simulink model "emulation_method"  (R2020b)
settings: Solver=ode45  StartTime=0.0  StopTime=5  FixedStep=0.0001  RelTol=1e-3
undefined symbols (not defined in the file): ctrl, daq, degs2rpm, denHwa, denHws, DiscIntNeverNeededParam, drv, gbox, K_w, mld, mot, numHwa, numHws, rads2rpm, sens, step_size, T, tau_hat, Tl
settings Model: Creator=gioel  LastModifiedBy=gioel
settings DataIOCC: ReturnWorkspaceOutputs=off

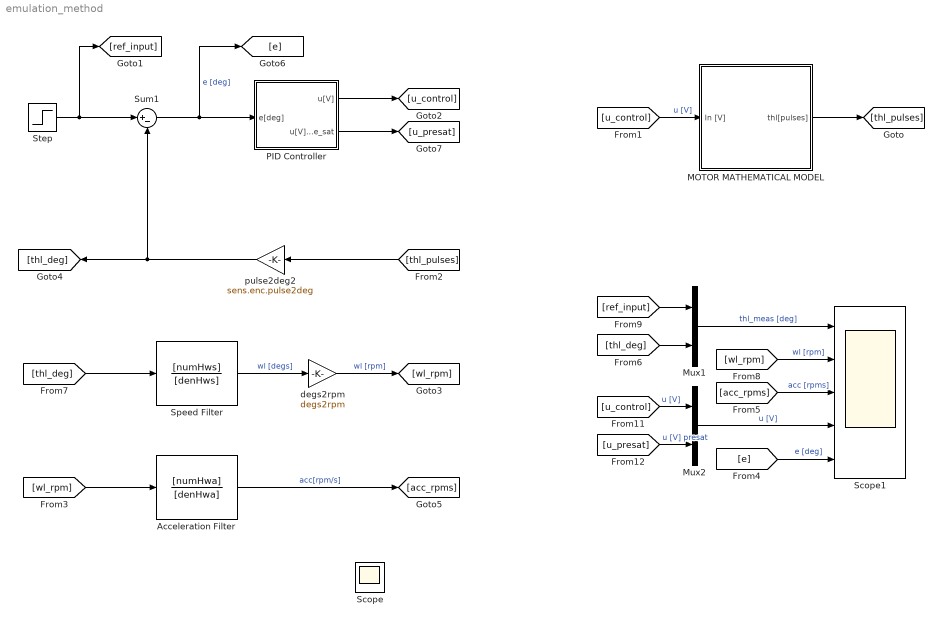
== system emulation_method ==
  Acceleration Filter : TransferFcn  Numerator=[numHwa]  Denominator=[denHwa]
  MOTOR MATHEMATICAL MODEL : Subsystem
  Mux1 : Mux  Inputs=2
  Mux2 : Mux  Inputs=2
  PID Controller : Subsystem
  Scope1 : Scope  NumInputPorts=5
  Speed Filter : TransferFcn  Numerator=[numHws]  Denominator=[denHws]
  Step : Step  After=step_size  SampleTime=0
  Sum1 : Sum  Inputs=|+-
  degs2rpm : Gain  Gain=degs2rpm
  pulse2deg2 : Gain  Gain=sens.enc.pulse2deg
  Scope : Scope
  wires:
  Sum1/1 -> [e], PID Controller/1(e[deg])  "e [deg]"
  Step/1 -> Sum1/1, [ref_input]
  PID Controller/1(u[V]) -> [u_control]
  Mux1/1 -> Scope1/1  "thl_meas [deg]"
  MOTOR MATHEMATICAL MODEL/1(thl[pulses]) -> [thl_pulses]
  degs2rpm/1 -> [wl_rpm]  "wl [rpm]"
  [thl_deg] -> Mux1/2
  [acc_rpms] -> Scope1/3  "acc [rpms]"
  [u_control] -> MOTOR MATHEMATICAL MODEL/1(In [V])  "u [V]"
  Mux2/1 -> Scope1/4  "u [V]"
  Speed Filter/1 -> degs2rpm/1  "wl [degs]"
  [wl_rpm] -> Scope1/2  "wl [rpm]"
  [wl_rpm] -> Acceleration Filter/1
  [thl_deg] -> Speed Filter/1
  [ref_input] -> Mux1/1
  Acceleration Filter/1 -> [acc_rpms]  "acc[rpm/s]"
  pulse2deg2/1 -> Sum1/2, [thl_deg]
  [thl_pulses] -> pulse2deg2/1
  [e] -> Scope1/5  "e [deg]"
  PID Controller/2(u[V] pre_sat) -> [u_presat]
  [u_control] -> Mux2/1  "u [V]"
  [u_presat] -> Mux2/2  "u [V] presat"

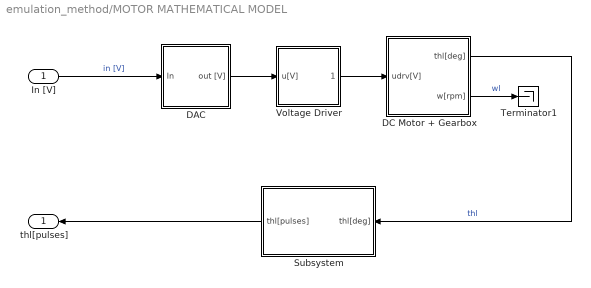
== system emulation_method/MOTOR MATHEMATICAL MODEL ==
  In [V] : Inport
  DAC : Subsystem
  DC Motor + Gearbox : Subsystem
  Subsystem : Subsystem
  Terminator1 : Terminator
  Voltage Driver : Subsystem
  thl[pulses] : Outport
  wires:
  In [V]/1 -> DAC/1(In)  "in [V]"
  DC Motor + Gearbox/1(thl[deg]) -> Subsystem/1(thl[deg])  "thl"
  DAC/1(out [V]) -> Voltage Driver/1(u[V])
  DC Motor + Gearbox/2(w[rpm]) -> Terminator1/1  "wl"
  Subsystem/1(thl[pulses]) -> thl[pulses]/1
  Voltage Driver/1(udrv[V]) -> DC Motor + Gearbox/1(udrv[V])

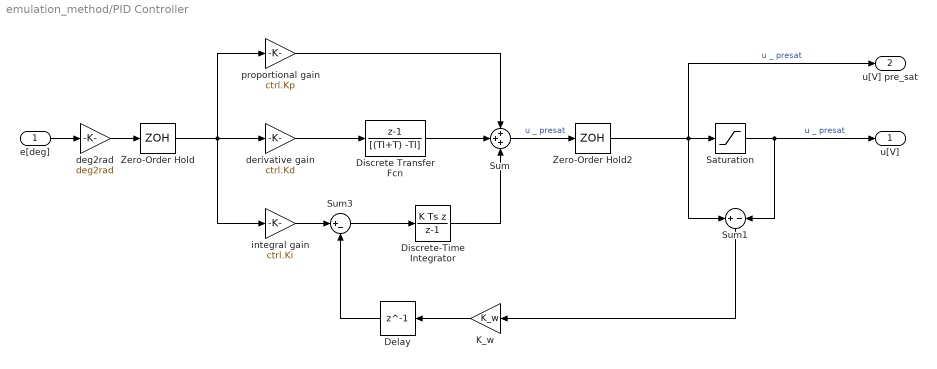
== system emulation_method/PID Controller ==
  e[deg] : Inport
  Delay : Delay  DelayLength=1  InitialCondition=0  SampleTime=T
  Discrete Transfer Fcn : DiscreteTransferFcn  Numerator=[1 -1]  Denominator=[(Tl+T) -Tl]  SampleTime=T
  Discrete-Time Integrator : DiscreteIntegrator  IntegratorMethod=Integration: Backward Euler  SampleTime=T  ICPrevOutput=DiscIntNeverNeededParam  ICPrevScaledInput=DiscIntNeverNeededParam
  "K_w " : Gain  Gain=K_w
  Saturation : Saturate  UpperLimit=10  LowerLimit=-10
  Sum : Sum  Inputs=+++
  Sum1 : Sum  Inputs=+|-
  Sum3 : Sum  Inputs=|+-
  Zero-Order Hold : ZeroOrderHold  SampleTime=T
  Zero-Order Hold2 : ZeroOrderHold  SampleTime=T
  deg2rad : Gain  Gain=deg2rad
  derivative gain : Gain  Gain=ctrl.Kd
  integral gain : Gain  Gain=ctrl.Ki
  proportional gain : Gain  Gain=ctrl.Kp
  u[V] : Outport
  u[V] pre_sat : Outport  Port=2
  wires:
  proportional gain/1 -> Sum/1
  e[deg]/1 -> deg2rad/1
  deg2rad/1 -> Zero-Order Hold/1
  Zero-Order Hold/1 -> integral gain/1, derivative gain/1, proportional gain/1
  derivative gain/1 -> Discrete Transfer Fcn/1
  Discrete Transfer Fcn/1 -> Sum/2
  Discrete-Time Integrator/1 -> Sum/3
  Sum1/1 -> "K_w "/1
  integral gain/1 -> Sum3/1
  Sum3/1 -> Discrete-Time Integrator/1
  "K_w "/1 -> Delay/1
  Delay/1 -> Sum3/2
  Sum/1 -> Zero-Order Hold2/1  "u _ presat"
  Saturation/1 -> u[V]/1, Sum1/2  "u _ presat"
  Zero-Order Hold2/1 -> u[V] pre_sat/1, Sum1/1, Saturation/1  "u _ presat"

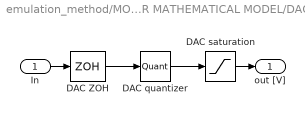
== system emulation_method/MOTOR MATHEMATICAL MODEL/DAC ==
  In : Inport
  DAC quantizer : Quantizer  QuantizationInterval=daq.dac.q
  DAC saturation : Saturate  UpperLimit=daq.dac.fs  LowerLimit=-daq.dac.fs
  DAC ZOH : ZeroOrderHold  SampleTime=0.001
  out [V] : Outport
  wires:
  DAC saturation/1 -> out [V]/1
  In/1 -> DAC ZOH/1
  DAC quantizer/1 -> DAC saturation/1
  DAC ZOH/1 -> DAC quantizer/1

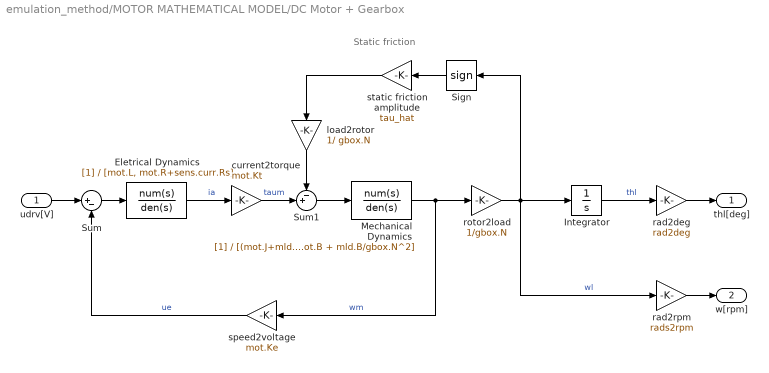
== system emulation_method/MOTOR MATHEMATICAL MODEL/DC Motor + Gearbox ==
  note: Static friction
  udrv[V] : Inport
  Eletrical Dynamics : TransferFcn  Denominator=[mot.L, mot.R+sens.curr.Rs]
  Integrator : Integrator
  Mechanical Dynamics : TransferFcn  Denominator=[(mot.J+mld.J/gbox.N^2), mot.B + mld.B/gbox.N^2]
  Sign : Signum  ZeroCross=off
  Sum : Sum  Inputs=|+-
  Sum1 : Sum  Inputs=-+|
  current2torque : Gain  Gain=mot.Kt
  load2rotor : Gain  Gain=1/ gbox.N
  rad2deg : Gain  Gain=rad2deg
  "rad2rpm " : Gain  Gain=rads2rpm
  rotor2load : Gain  Gain=1/gbox.N
  speed2voltage : Gain  Gain=mot.Ke
  static friction amplitude : Gain  Gain=tau_hat
  thl[deg] : Outport  VectorParamsAs1DForOutWhenUnconnected=off
  w[rpm] : Outport  Port=2  VectorParamsAs1DForOutWhenUnconnected=off
  wires:
  Eletrical Dynamics/1 -> current2torque/1  "ia"
  udrv[V]/1 -> Sum/1
  Sum/1 -> Eletrical Dynamics/1
  current2torque/1 -> Sum1/2  "taum"
  Sum1/1 -> Mechanical Dynamics/1
  Mechanical Dynamics/1 -> rotor2load/1, speed2voltage/1  "wm"
  rotor2load/1 -> Integrator/1, "rad2rpm "/1, Sign/1  "wl"
  Integrator/1 -> rad2deg/1  "thl"
  rad2deg/1 -> thl[deg]/1
  "rad2rpm "/1 -> w[rpm]/1
  Sign/1 -> static friction amplitude/1
  speed2voltage/1 -> Sum/2  "ue"
  static friction amplitude/1 -> load2rotor/1
  load2rotor/1 -> Sum1/1

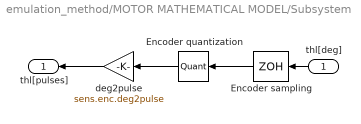
== system emulation_method/MOTOR MATHEMATICAL MODEL/Subsystem ==
  thl[deg] : Inport
  Encoder quantization : Quantizer  QuantizationInterval=sens.enc.pulse2deg
  Encoder sampling : ZeroOrderHold  SampleTime=-1
  deg2pulse : Gain  Gain=sens.enc.deg2pulse
  thl[pulses] : Outport
  wires:
  thl[deg]/1 -> Encoder sampling/1
  Encoder quantization/1 -> deg2pulse/1
  Encoder sampling/1 -> Encoder quantization/1
  deg2pulse/1 -> thl[pulses]/1

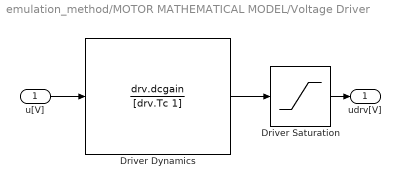
== system emulation_method/MOTOR MATHEMATICAL MODEL/Voltage Driver ==
  u[V] : Inport
  Driver Dynamics : TransferFcn  Numerator=drv.dcgain  Denominator=[drv.Tc 1]
  Driver Saturation : Saturate  UpperLimit=12  LowerLimit=-12
  udrv[V] : Outport
  wires:
  u[V]/1 -> Driver Dynamics/1
  Driver Saturation/1 -> udrv[V]/1
  Driver Dynamics/1 -> Driver Saturation/1
